simulink model "vtol_lon_inner_q"  (R2024b)
settings: Solver=VariableStepAuto  StartTime=0.0  StopTime=10.0  RelTol=1e-3
undefined symbols (not defined in the file or in its folder): A_vtol_lon, B_vtol_lon, C_vtol_lon, D_vtol_lon, Ki_q, Kp_q
libraries: simulink x1
settings Model: Creator=mhcho  LastModifiedBy=mhcho

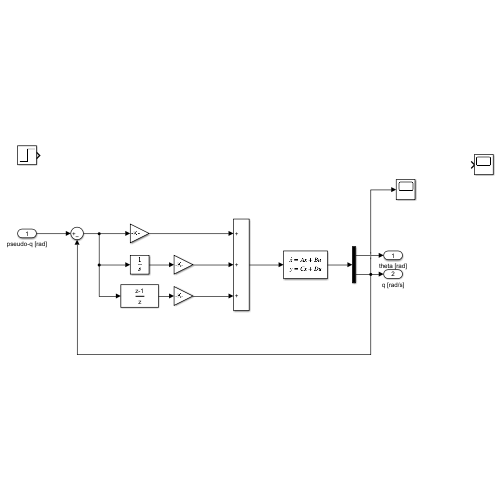
[thumbnail: Simulink's stored preview of the top-level diagram]
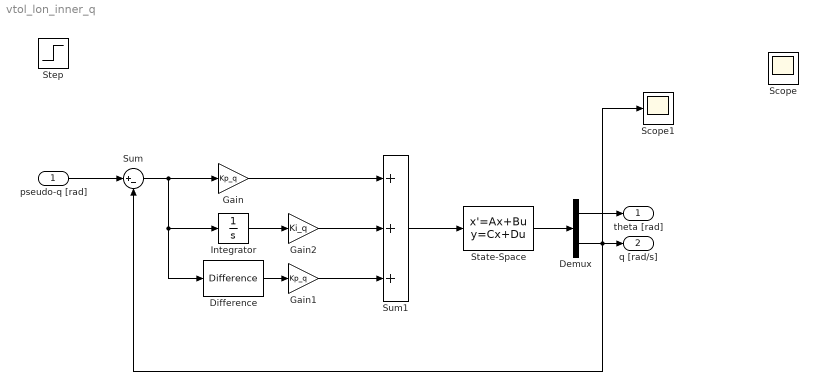
== system vtol_lon_inner_q ==
  pseudo-q [rad] : Inport
  Demux : Demux  Outputs=2
  Difference : simulink/Discrete/Difference  ICPrevInput=0.0  OutMin=[]  OutMax=[]  OutDataType=fixdt(1, 16)  OutScaling=2^-10  DoSatur=off
  Gain : Gain  Gain=Kp_q
  Gain1 : Gain  Gain=Kp_q
  Gain2 : Gain  Gain=Ki_q
  Integrator : Integrator
  Scope : Scope
  Scope1 : Scope
  State-Space : StateSpace  A=A_vtol_lon(3:4,3:4)  B=B_vtol_lon(3:4,1)  C=C_vtol_lon(3:4,3:4)  D=D_vtol_lon(3:4,1)  InitialCondition=0
  Step : Step  SampleTime=0
  Sum : Sum  Inputs=|+-
  Sum1 : Sum  Inputs=+++
  theta [rad] : Outport
  q [rad/s] : Outport  Port=2
  wires:
  State-Space/1 -> Demux/1
  Demux/1 -> theta [rad]/1
  Demux/2 -> Scope1/1, Sum/2, q [rad/s]/1
  Sum/1 -> Difference/1, Integrator/1, Gain/1
  Difference/1 -> Gain1/1
  Integrator/1 -> Gain2/1
  Gain/1 -> Sum1/1
  Gain2/1 -> Sum1/2
  Gain1/1 -> Sum1/3
  Sum1/1 -> State-Space/1
  pseudo-q [rad]/1 -> Sum/1
